simulink model "ac_ac_controller"  (R2020a)
settings: Solver=VariableStepAuto  StartTime=0.0  StopTime=inf  RelTol=1e-3
libraries: powerlib x7, powerlib_meascontrol x2
settings Model: Creator=snehk  LastModifiedBy=snehk

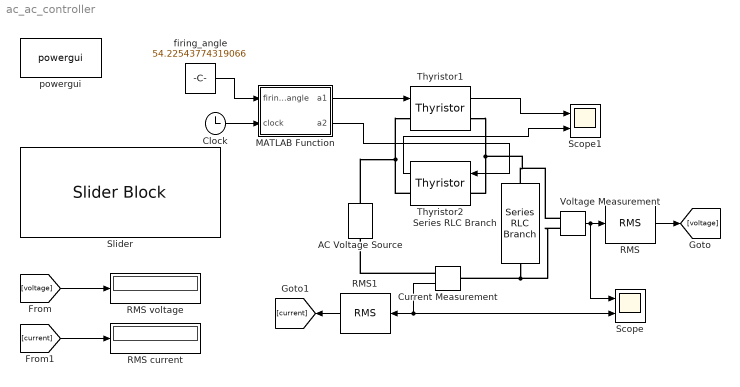
== system ac_ac_controller ==
  AC Voltage Source : powerlib/Electrical Sources/AC Voltage Source  Amplitude=230  Phase=0  Frequency=50  SampleTime=0  Measurements=None  BusType=swing  Pref=10e3  Qref=0  Qmin=-inf  Qmax=+inf
  Clock : Clock
  Current Measurement : powerlib/Measurements/Current Measurement  PhasorSimulation=off  OutputType=Complex  PSBequivalent=0
  MATLAB Function : MATLAB Function  TreatAsAtomicUnit=on
  RMS : powerlib_meascontrol/Measurements/RMS  TrueRMS=on  Freq=50  RMSInit=0  Ts=0
  RMS current : Display
  RMS voltage : Display
  RMS1 : powerlib_meascontrol/Measurements/RMS  TrueRMS=on  Freq=50  RMSInit=0  Ts=0
  Scope : Scope  NumInputPorts=2
  Scope1 : Scope  NumInputPorts=2
  Series RLC Branch : powerlib/Elements/Series RLC Branch  LConnTagsString=__new0  RConnTagsString=__new0  BranchType=RL  Resistance=100  Inductance=100e-3  SetiL0=off  InitialCurrent=0  Capacitance=1e-6  Setx0=off  InitialVoltage=0  Measurements=None
  Slider : SliderBlock  LabelPosition=Bottom  ScaleMax=180
  Thyristor1 : powerlib/Power Electronics/Thyristor  Ron=0  Lon=0  Vf=0  IC=0  Rs=500  Cs=250e-9  Measurements=on
  Thyristor2 : powerlib/Power Electronics/Thyristor  Ron=0  Lon=0  Vf=0  IC=0  Rs=500  Cs=250e-9  Measurements=on
  Voltage Measurement : powerlib/Measurements/Voltage Measurement  PhasorSimulation=off  OutputType=Complex  PSBequivalent=0
  firing_angle : Constant  Value=54.22543774319066
  powergui : powerlib/powergui  Priority=1  SimulationMode=Continuous  SampleTime=50e-6  frequency=60  Iterations=50  frequencyindice=50  Pbase=100e6  ErrMax=1e-4  UnitsV=kV  UnitsW=MW  buscounter=0  FunctionMessages=off  echomessages=off  EnableUseOfTLC=off  CurrentSourceSwitches=off  DisableSnubberDevices=off  DisableRonSwitches=off  DisableVfSwitches=off  DisplayEquations=off  AutomaticDiscreteSolvers=off  SolverType=Tustin/Backward Euler (TBE)  Interpol=off  ExternalGateDelay=off  methode=off  Ts=100  x0status=blocks  SPID=on  SwTol=0  HookPort=off  NonlinearTolerance=1e-4  nMaxIteration=100  ContinueOnMaxIteration=off  RestoreLinks=warning  ResistiveCurrentMeasurement=off  Frange=[0:2:500]  Ylog=off  Xlog=on  ShowGrid=off  save=off  variable=ZData  structure=0  ZoomFFT=off  StartTime=0.0  cycles=1  DisplayStyle=1  fundamental=60  FreqAxis=off  MaxFrequency=1000  frequencyindicesteady=1  RmsSteady=1  display=off
  wires:
  MATLAB Function/1(a1) -> Thyristor1/1
  MATLAB Function/2(a2) -> Thyristor2/1
  Clock/1 -> MATLAB Function/2(clock)
  firing_angle/1 -> MATLAB Function/1(firing_angle)
  Voltage Measurement/1 -> Scope/1, RMS/1
  Current Measurement/1 -> Scope/2, RMS1/1
  RMS1/1 -> [current]
  RMS/1 -> [voltage]
  [voltage] -> RMS voltage/1
  [current] -> RMS current/1
  Thyristor1/1 -> Scope1/1
  Thyristor2/1 -> Scope1/2
  connections:
  Thyristor2/RConn1 -- AC Voltage Source/RConn1 -- Thyristor1/LConn1
  Thyristor1/RConn1 -- Voltage Measurement/LConn1 -- Series RLC Branch/LConn1 -- Thyristor2/LConn1
  Series RLC Branch/RConn1 -- Current Measurement/LConn1 -- Voltage Measurement/LConn2
  Current Measurement/RConn1 -- AC Voltage Source/LConn1

== matlab function ac_ac_controller/MATLAB Function ==
  data: firing_angle input; a1 output; a2 output; clock input
function [a1, a2] = fcn(firing_angle, clock)
f = 50;

tt1 = 1/(2*f);

t = mod(clock,(1/(f)));
a = firing_angle/180;
if (t < (tt1))
    if (t > (a*tt1))
        a1 = 1;
        a2 = 0;
    else
        a1 = 0;
        a2 = 0;
    end
else 
    if (t > (a/f))
        a2 = 1;
        a1 = 0; 
    else
        a1 = 0;
        a2 = 0;
    end
end
